simulink model "sis5"  (Simulink 8.0)
settings: Solver=ode45  StartTime=0.0  StopTime=20  RelTol=1e-9
values from neighbouring files (symbols this model uses):
  k = [10]    [Laboratorio2.m]
libraries: simulink x1
settings Model: Creator=Katarina  LastModifiedBy=Katarina
settings DataIOCC: LimitDataPoints=off
settings DebuggingCC: SolverPrmCheckMsg=none  FcnCallInpInsideContextMsg=UseLocalSettings
settings GRTTargetCC: CombineOutputUpdateFcns=off  GRTInterface=on

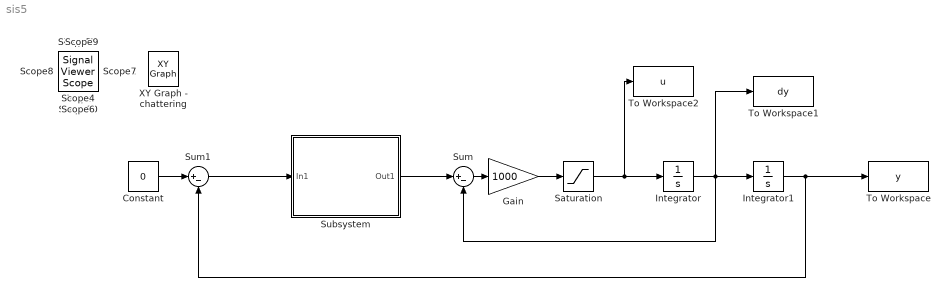
== system sis5 ==
  Constant : Constant  Value=0
  Gain : Gain  Gain=1000
  Integrator : Integrator
  Integrator1 : Integrator  InitialCondition=k
  Saturation : Saturate  UpperLimit=1  LowerLimit=-1
  Subsystem : Subsystem
  Sum : Sum  Inputs=|+-
  Sum1 : Sum  Inputs=|+-
  To Workspace : ToWorkspace  VariableName=y  SampleTime=-1
  To Workspace1 : ToWorkspace  VariableName=dy  SampleTime=-1
  To Workspace2 : ToWorkspace  VariableName=u  SampleTime=-1
  Scope{,3,5..10} (8 alike) : SignalViewerScope  IOType=viewer  RefreshTime=0.035000
      Scope10 settings: SaveName=ScopeData10
      Scope3 settings: SaveName=ScopeData3
      Scope5 settings: SaveName=ScopeData5
      Scope6 settings: SaveName=ScopeData6
      Scope7 settings: SaveName=ScopeData7
      Scope8 settings: SaveName=ScopeData8
      Scope9 settings: SaveName=ScopeData9
  Scope1 : SignalViewerScope  IOType=viewer  ZoomMode=yonly  RefreshTime=0.035000
  Scope2 : SignalViewerScope  IOType=viewer  ZoomMode=yonly  RefreshTime=0.035000
      settings: SaveName=ScopeData2
  Scope4 : SignalViewerScope  IOType=viewer  ZoomMode=yonly  RefreshTime=0.035000
      settings: SaveName=ScopeData4
  XY Graph - chattering : simulink/Sinks/XY Graph  IOType=viewer  xmin=xmin  xmax=xmax  ymin=ymin  ymax=ymax  st=-1
  wires:
  Integrator1/1 -> To Workspace/1, Sum1/2
  Integrator/1 -> To Workspace1/1, Sum/2, Integrator1/1
  Saturation/1 -> To Workspace2/1, Integrator/1
  Gain/1 -> Saturation/1
  Subsystem/1(Out1) -> Sum/1
  Sum/1 -> Gain/1
  Constant/1 -> Sum1/1
  Sum1/1 -> Subsystem/1(In1)

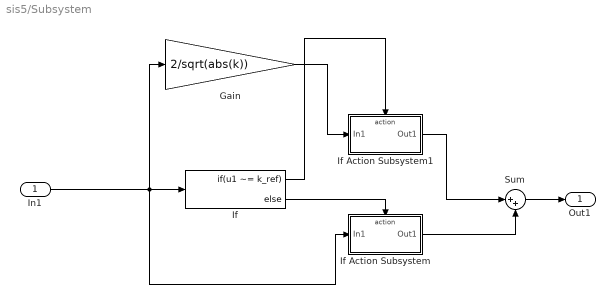
== system sis5/Subsystem ==
  In1 : Inport
  Gain : Gain  Gain=2/sqrt(abs(k))
  If : If  IfExpression=u1 ~= k_ref
  If Action Subsystem : Subsystem  TreatAsAtomicUnit=on
  If Action Subsystem1 : Subsystem  TreatAsAtomicUnit=on
  Sum : Sum  Inputs=|++
  Out1 : Outport
  wires:
  In1/1 -> If/1, If Action Subsystem/1(In1), Gain/1
  If/2 -> If Action Subsystem/Action
  Sum/1 -> Out1/1
  If/1 -> If Action Subsystem1/Action
  Gain/1 -> If Action Subsystem1/1(In1)
  If Action Subsystem1/1(Out1) -> Sum/1
  If Action Subsystem/1(Out1) -> Sum/2

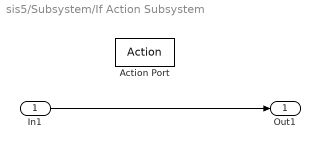
== system sis5/Subsystem/If Action Subsystem ==
  In1 : Inport
  Action Port : ActionPort  ActionType=else
  Out1 : Outport
  wires:
  In1/1 -> Out1/1

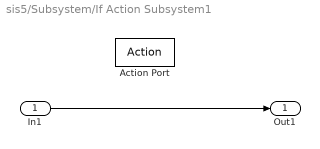
== system sis5/Subsystem/If Action Subsystem1 ==
  In1 : Inport
  Action Port : ActionPort  ActionType=then
  Out1 : Outport
  wires:
  In1/1 -> Out1/1
